simulink model "problem_4"  (R2020b)
settings: Solver=VariableStepAuto  StartTime=0.0  StopTime=10.0  RelTol=1e-3
settings Model: Creator=sonal  LastModifiedBy=sonal

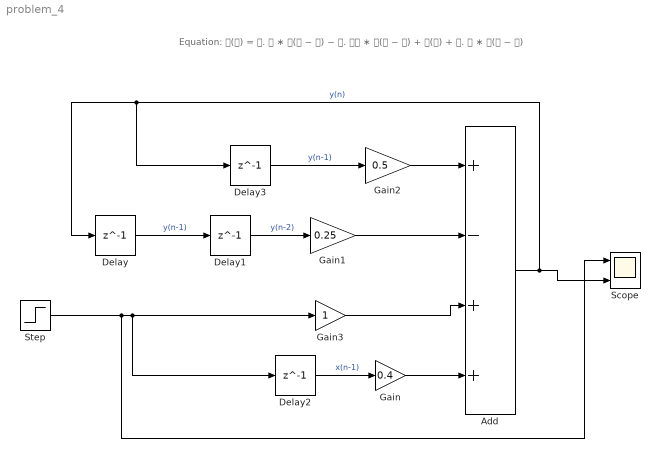
== system problem_4 ==
  note: Equation: 𝐲(𝐧) = 𝟎. 𝟓 ∗ 𝐲(𝐧 − 𝟏) − 𝟎. 𝟐𝟓 ∗ 𝐲(𝐧 − 𝟐) + 𝐱(𝐧) + 𝟎. 𝟒 ∗ 𝐱(𝐧 − 𝟏)
  Add : Sum  Inputs=+-++
  Delay{,1..3} (4 alike) : Delay  DelayLength=1
  Gain : Gain  Gain=0.4
  Gain1 : Gain  Gain=0.25
  Gain2 : Gain  Gain=0.5
  Gain3 : Gain
  Scope : Scope  NumInputPorts=2
  Step : Step  SampleTime=0
  wires:
  Delay2/1 -> Gain/1  "x(n-1)"
  Delay/1 -> Delay1/1  "y(n-1)"
  Gain1/1 -> Add/2
  Delay3/1 -> Gain2/1  "y(n-1)"
  Gain/1 -> Add/4
  Gain2/1 -> Add/1
  Gain3/1 -> Add/3
  Delay1/1 -> Gain1/1  "y(n-2)"
  Step/1 -> Scope/1, Delay2/1, Gain3/1
  Add/1 -> Delay3/1, Delay/1, Scope/2  "y(n)"
